simulink model "OpenLoop_1"  (R2016b)
settings: Solver=VariableStepAuto  StartTime=0.0  StopTime=10.0  RelTol=1e-3
values from neighbouring files (symbols this model uses):
  A = [0 0 1 0; 0 0 0 1; -k/J1 k/J1 -c/J1 c/J1; k/J2 -k/J2 c/J2 -c/J2]    [ELEC341Project.m]    (also in Question6and8.m)
  BI = [0; 0; kI/J1; 0]    [Question6and8.m]
  BTd = [0; 0; 0; 1/J2]    [Question6and8.m]
  C = [0 1 0 0]    [ELEC341Project.m]    (also in Question6and8.m)
settings Model: Creator=isaacjacobsen  LastModifiedBy=isaacjacobsen

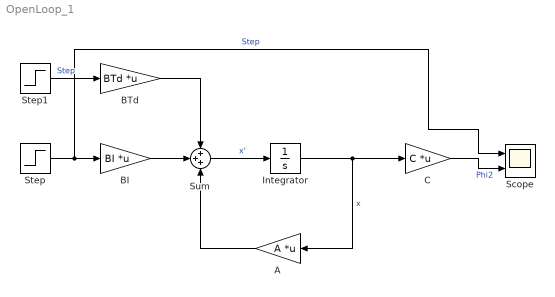
== system OpenLoop_1 ==
  A : Gain  Gain=A  Multiplication=Matrix(K*u)
  BI : Gain  Gain=BI  Multiplication=Matrix(K*u)
  BTd : Gain  Gain=BTd  Multiplication=Matrix(K*u)
  C : Gain  Gain=C  Multiplication=Matrix(K*u)
  Integrator : Integrator
  Scope : Scope  NumInputPorts=2
  Step : Step  Time=0  SampleTime=0
  Step1 : Step  Time=0  SampleTime=0
  Sum : Sum  Inputs=+++
  wires:
  Sum/1 -> Integrator/1  "x'"
  Integrator/1 -> A/1, C/1  "x"
  A/1 -> Sum/3
  BI/1 -> Sum/2
  BTd/1 -> Sum/1
  Step/1 -> Scope/1, BI/1  "Step"
  C/1 -> Scope/2  "Phi2"
  Step1/1 -> BTd/1  "Step"
